simulink model "NOLCO3"  (R2017b)
settings: Solver=ode1  StartTime=0.0  StopTime=20.0  FixedStep=0.0001  RelTol=1e-3
values from neighbouring files (symbols this model uses):
  lamda = [30 300 1000]    [config3.m]
settings Model: Creator=lbergantin2017  LastModifiedBy=miche
settings CodeAppCC: StateflowObjectComments=on

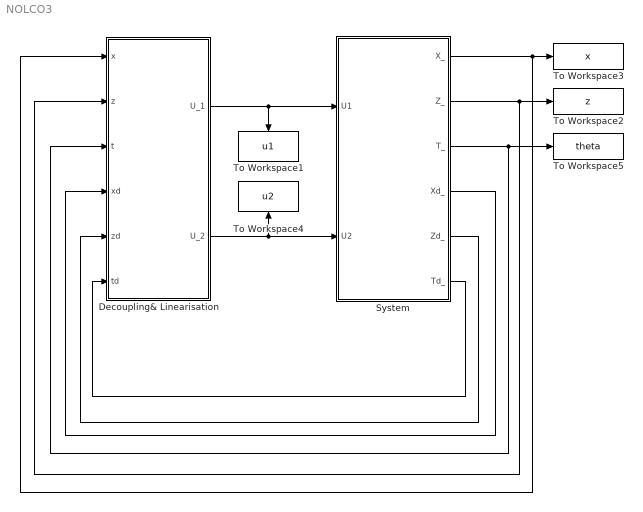
== system NOLCO3 ==
  Decoupling& Linearisation : Subsystem
  System : Subsystem
  To Workspace1 : ToWorkspace  VariableName=u1  SampleTime=-1
  To Workspace2 : ToWorkspace  VariableName=z  SampleTime=-1
  To Workspace3 : ToWorkspace  VariableName=x  SampleTime=-1
  To Workspace4 : ToWorkspace  VariableName=u2  SampleTime=-1
  To Workspace5 : ToWorkspace  VariableName=theta  SampleTime=-1
  wires:
  Decoupling& Linearisation/1(U_1) -> To Workspace1/1, System/1("U1 ")
  System/1(X_) -> To Workspace3/1, Decoupling& Linearisation/1(x)
  System/2("Z_ ") -> Decoupling& Linearisation/2(z), To Workspace2/1
  Decoupling& Linearisation/2(U_2) -> System/2(U2), To Workspace4/1
  System/3(T_) -> Decoupling& Linearisation/3("t "), To Workspace5/1
  System/4(Xd_) -> Decoupling& Linearisation/4(xd)
  System/5(Zd_) -> Decoupling& Linearisation/5(zd)
  System/6(Td_) -> Decoupling& Linearisation/6(td)

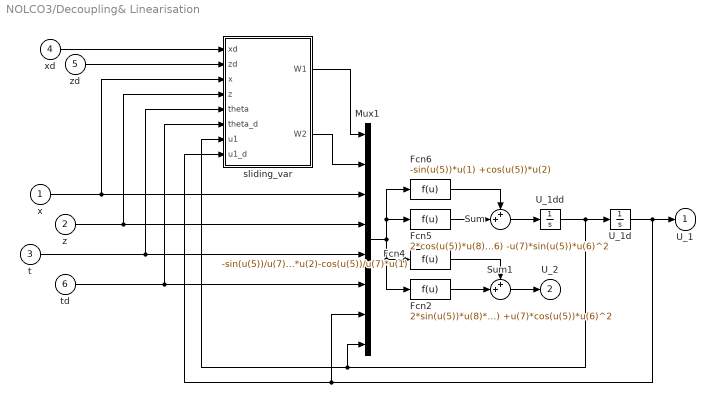
== system NOLCO3/Decoupling& Linearisation ==
  x : Inport
  z : Inport  Port=2
  "t " : Inport  Port=3
  xd : Inport  Port=4
  zd : Inport  Port=5
  td : Inport  Port=6
  Fcn2 : Fcn  Expr=2*sin(u(5))*u(8)*u(6) +u(7)*cos(u(5))*u(6)^2
  Fcn4 : Fcn  Expr=-sin(u(5))/u(7)*u(2)-cos(u(5))/u(7)*u(1)
  Fcn5 : Fcn  Expr=2*cos(u(5))*u(8)*u(6) -u(7)*sin(u(5))*u(6)^2
  Fcn6 : Fcn  Expr=-sin(u(5))*u(1) +cos(u(5))*u(2)
  Mux1 : Mux  Inputs=8
  Sum : Sum  Inputs=++|
  Sum1 : Sum  Inputs=++|
  U_1d : Integrator  InitialCondition=1
  U_1dd : Integrator
  sliding_var : Subsystem
  U_1 : Outport
  U_2 : Outport  Port=2
  wires:
  x/1 -> sliding_var/3(x), Mux1/3
  "t "/1 -> sliding_var/5(theta), Mux1/5
  Mux1/1 -> Fcn2/1, Fcn4/1, Fcn5/1, Fcn6/1
  z/1 -> sliding_var/4(z), Mux1/4
  Fcn6/1 -> Sum/1
  Fcn5/1 -> Sum/2
  td/1 -> Mux1/6, sliding_var/6(theta_d)
  Sum/1 -> U_1dd/1
  U_1dd/1 -> sliding_var/7(u1), Mux1/8, U_1d/1
  U_1d/1 -> sliding_var/8(u1_d), Mux1/7, U_1/1
  Sum1/1 -> U_2/1
  Fcn2/1 -> Sum1/2
  Fcn4/1 -> Sum1/1
  xd/1 -> sliding_var/1(xd)
  zd/1 -> sliding_var/2(zd)
  sliding_var/1(W1) -> Mux1/1
  sliding_var/2(W2) -> Mux1/2

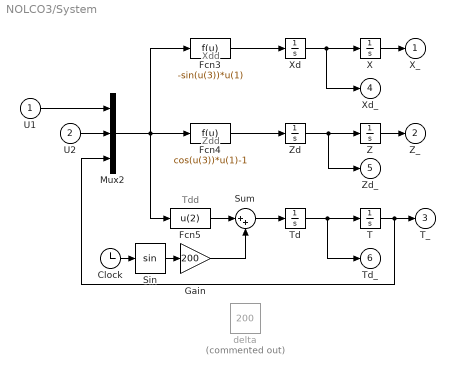
== system NOLCO3/System ==
  note: Xdd
  note: Zdd
  note: Tdd
  "U1 " : Inport
  U2 : Inport  Port=2
  Clock : Clock
  Fcn3 : Fcn  Expr=-sin(u(3))*u(1)
  Fcn4 : Fcn  Expr=cos(u(3))*u(1)-1
  Fcn5 : Fcn  Expr=u(2)
  Gain : Gain  Gain=200
  Mux2 : Mux  Inputs=3
  Sin : Trigonometry
  Sum : Sum  Inputs=|++
  T : Integrator  InitialCondition=1
  Td : Integrator  InitialCondition=1
  X : Integrator  InitialCondition=1
  Xd : Integrator
  Z : Integrator  InitialCondition=1
  Zd : Integrator
  delta : Constant  Commented=on  Value=200
  X_ : Outport
  "Z_ " : Outport  Port=2
  T_ : Outport  Port=3
  Xd_ : Outport  Port=4
  Zd_ : Outport  Port=5
  Td_ : Outport  Port=6
  wires:
  Fcn3/1 -> Xd/1
  Xd/1 -> Xd_/1, X/1
  Zd/1 -> Zd_/1, Z/1
  Fcn4/1 -> Zd/1
  Mux2/1 -> Fcn5/1, Fcn3/1, Fcn4/1
  Td/1 -> Td_/1, T/1
  "U1 "/1 -> Mux2/1
  U2/1 -> Mux2/2
  X/1 -> X_/1
  Z/1 -> "Z_ "/1
  T/1 -> T_/1, Mux2/3
  Sum/1 -> Td/1
  Fcn5/1 -> Sum/1
  Clock/1 -> Sin/1
  Sin/1 -> Gain/1
  Gain/1 -> Sum/2

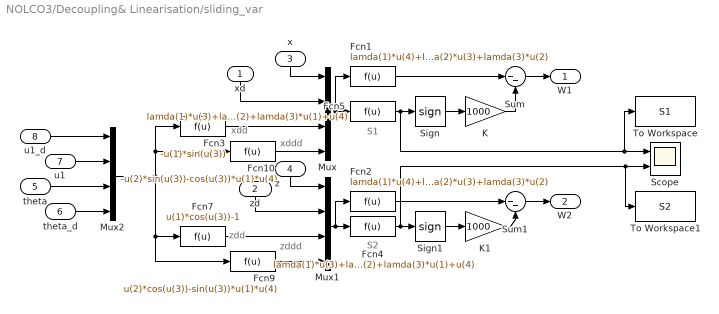
== system NOLCO3/Decoupling& Linearisation/sliding_var ==
  note: S1
  note: zddd
  note: xddd
  note: xdd
  note: zdd
  note: S2
  xd : Inport
  zd : Inport  Port=2
  x : Inport  Port=3
  z : Inport  Port=4
  theta : Inport  Port=5
  theta_d : Inport  Port=6
  u1 : Inport  Port=7
  u1_d : Inport  Port=8
  Fcn1 : Fcn  Expr=lamda(1)*u(4)+lamda(2)*u(3)+lamda(3)*u(2)
  Fcn10 : Fcn  Expr=-u(2)*sin(u(3))-cos(u(3))*u(1)*u(4)
  Fcn2 : Fcn  Expr=lamda(1)*u(4)+lamda(2)*u(3)+lamda(3)*u(2)
  Fcn3 : Fcn  Expr=-u(1)*sin(u(3))
  Fcn4 : Fcn  Expr=lamda(1)*u(3)+lamda(2)*u(2)+lamda(3)*u(1)+u(4)
  Fcn5 : Fcn  Expr=lamda(1)*u(3)+lamda(2)*u(2)+lamda(3)*u(1)+u(4)
  Fcn7 : Fcn  Expr=u(1)*cos(u(3))-1
  Fcn9 : Fcn  Expr=u(2)*cos(u(3))-sin(u(3))*u(1)*u(4)
  K : Gain  Gain=1000
  K1 : Gain  Gain=1000
  Mux : Mux
  Mux1 : Mux
  Mux2 : Mux
  Scope : Scope  NumInputPorts=2
  Sign : Signum
  Sign1 : Signum
  Sum : Sum  Inputs=|--
  Sum1 : Sum  Inputs=|--
  To Workspace : ToWorkspace  VariableName=S1  SampleTime=-1
  To Workspace1 : ToWorkspace  VariableName=S2  SampleTime=-1
  W1 : Outport
  W2 : Outport  Port=2
  wires:
  xd/1 -> Mux/2
  u1_d/1 -> Mux2/1
  x/1 -> Mux/1
  Fcn3/1 -> Mux/3
  Fcn7/1 -> Mux1/3
  zd/1 -> Mux1/2
  Mux/1 -> Fcn5/1, Fcn1/1
  theta/1 -> Mux2/3
  u1/1 -> Mux2/2
  theta_d/1 -> Mux2/4
  z/1 -> Mux1/1
  Mux2/1 -> Fcn3/1, Fcn10/1, Fcn7/1, Fcn9/1
  Sum1/1 -> W2/1
  Fcn10/1 -> Mux/4
  Fcn9/1 -> Mux1/4
  Sum/1 -> W1/1
  Mux1/1 -> Fcn4/1, Fcn2/1
  Fcn4/1 -> To Workspace1/1, Scope/2, Sign1/1
  Sign/1 -> K/1
  K/1 -> Sum/2
  Sign1/1 -> K1/1
  K1/1 -> Sum1/2
  Fcn1/1 -> Sum/1
  Fcn2/1 -> Sum1/1
  Fcn5/1 -> To Workspace/1, Scope/1, Sign/1
